simulink model "dronePID"  (R2018b)
settings: Solver=VariableStepAuto  StartTime=0.0  StopTime=10  RelTol=1e-3
libraries: simulink x3
settings Model: Creator=vietdo  LastModifiedBy=Viet Do

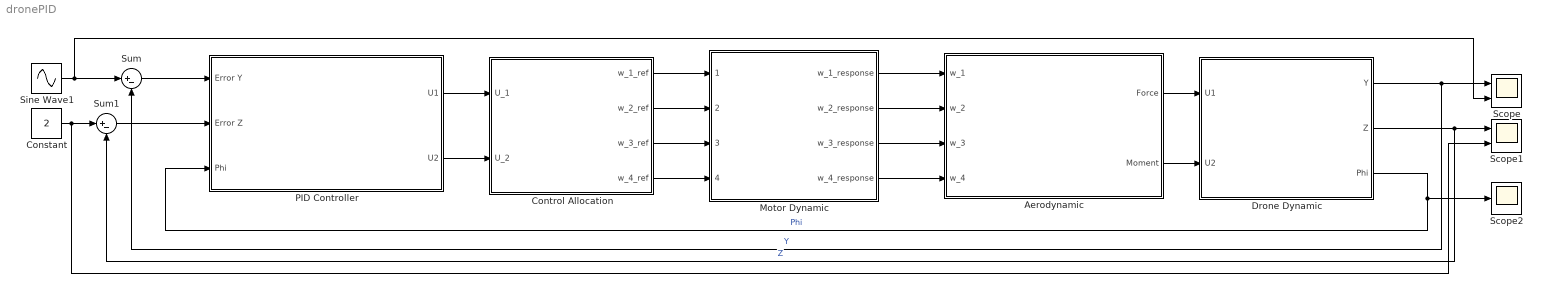
== system dronePID ==
  Aerodynamic : Subsystem  mask{b=2.980e-6, l=0.225}
      mask prompts: b "Lift Constant"; l "Distance between the rotor and the center of mass (m)"
      mask Display: image('blade.png');
  Constant : Constant  Value=2
  Control Allocation : Subsystem  mask{b=2.980e-6, l=0.225}
      mask prompts: b "Lift Constant"; l "Distance between rotor and the center of mass (m)"
      mask Display: image('incsl.png');
  Drone Dynamic : Subsystem  mask{m=0.468, Ixx=4.856e-3, g=9.81}
      mask prompts: m "Mass(kg)"; Ixx "Inertia Moment (kg.m^2)"; g "Gravity(m/s^2)"
      mask Display: image('drone.jpg');
  Motor Dynamic : Subsystem
      mask Display: image('motor.jpg');
  PID Controller : Subsystem
      mask Display: image('PID.png');
  Scope : Scope  NumInputPorts=2
  Scope1 : Scope  NumInputPorts=2
  Scope2 : Scope
  Sine Wave1 : Sin  Frequency=0.2  SampleTime=0
  Sum : Sum  Inputs=|+-
  Sum1 : Sum  Inputs=|+-
  wires:
  Drone Dynamic/1(Y) -> Scope/1, Sum/2  "Y"
  Drone Dynamic/2(Z) -> Scope1/1, Sum1/2  "Z"
  Drone Dynamic/3("Phi ") -> PID Controller/3(Phi), Scope2/1  "Phi"
  Sum/1 -> PID Controller/1(Error Y)
  Sum1/1 -> PID Controller/2(Error Z)
  Sine Wave1/1 -> Scope/2, Sum/1
  Constant/1 -> Scope1/2, Sum1/1
  PID Controller/1(U1) -> Control Allocation/1(U_1)
  PID Controller/2(U2) -> Control Allocation/2(U_2)
  Aerodynamic/1(Force) -> Drone Dynamic/1(U1)
  Aerodynamic/2(Moment) -> Drone Dynamic/2(U2)
  Control Allocation/1(w_1_ref) -> Motor Dynamic/1(1)
  Control Allocation/2(w_2_ref) -> Motor Dynamic/2(2)
  Control Allocation/3(w_3_ref) -> Motor Dynamic/3(3)
  Control Allocation/4(w_4_ref) -> Motor Dynamic/4(4)
  Motor Dynamic/1(w_1_response) -> Aerodynamic/1(w_1)
  Motor Dynamic/2(w_2_response) -> Aerodynamic/2(w_2)
  Motor Dynamic/3(w_3_response) -> Aerodynamic/3(w_3)
  Motor Dynamic/4(w_4_response) -> Aerodynamic/4(w_4)

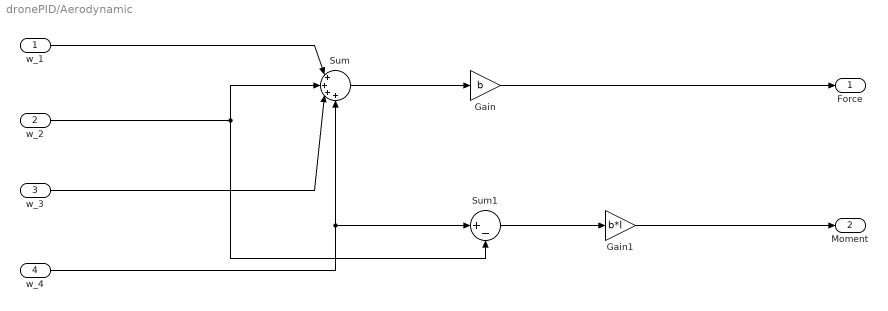
== system dronePID/Aerodynamic ==
  w_1 : Inport
  w_2 : Inport  Port=2
  w_3 : Inport  Port=3
  w_4 : Inport  Port=4
  Gain : Gain  Gain=b
  Gain1 : Gain  Gain=b*l
  Sum : Sum  Inputs=|++++
  Sum1 : Sum  Inputs=|+-
  Force : Outport
  Moment : Outport  Port=2
  wires:
  Sum/1 -> Gain/1
  Gain/1 -> Force/1
  Gain1/1 -> Moment/1
  Sum1/1 -> Gain1/1
  w_1/1 -> Sum/1
  w_2/1 -> Sum1/2, Sum/2
  w_3/1 -> Sum/3
  w_4/1 -> Sum1/1, Sum/4

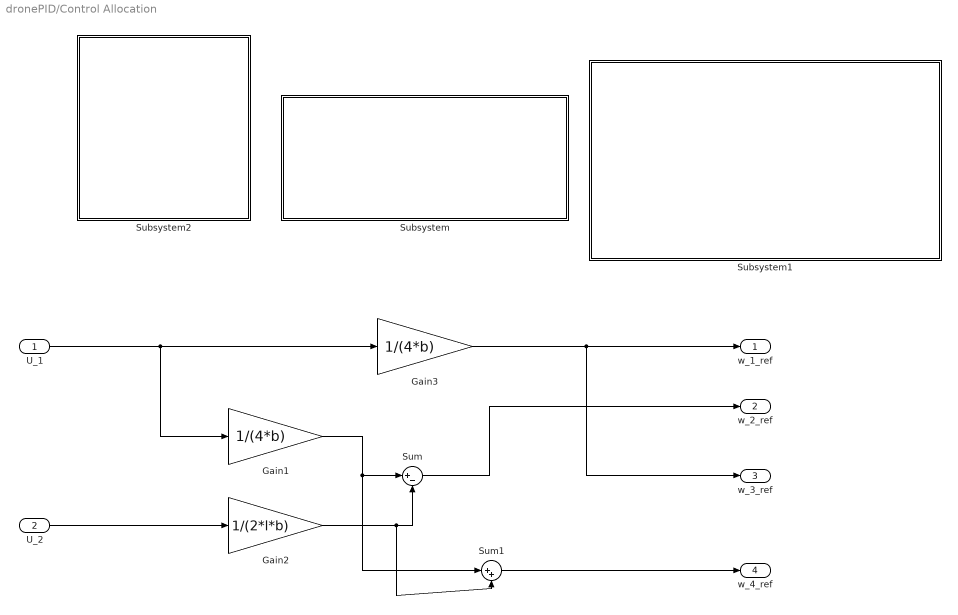
== system dronePID/Control Allocation ==
  U_1 : Inport
  U_2 : Inport  Port=2
  Gain1 : Gain  Gain=1/(4*b)
  Gain2 : Gain  Gain=1/(2*l*b)
  Gain3 : Gain  Gain=1/(4*b)
  Subsystem : Subsystem
      mask Display: image('allocation_1.png');
  Subsystem1 : Subsystem
      mask Display: image('allocation_2.png');
  Subsystem2 : Subsystem
      mask Display: image('allocation_3.png');
  Sum : Sum  Inputs=|+-
  Sum1 : Sum  Inputs=|++
  w_1_ref : Outport
  w_2_ref : Outport  Port=2
  w_3_ref : Outport  Port=3
  w_4_ref : Outport  Port=4
  wires:
  U_1/1 -> Gain3/1, Gain1/1
  Gain1/1 -> Sum1/1, Sum/1
  Gain2/1 -> Sum1/2, Sum/2
  U_2/1 -> Gain2/1
  Gain3/1 -> w_1_ref/1, w_3_ref/1
  Sum/1 -> w_2_ref/1
  Sum1/1 -> w_4_ref/1

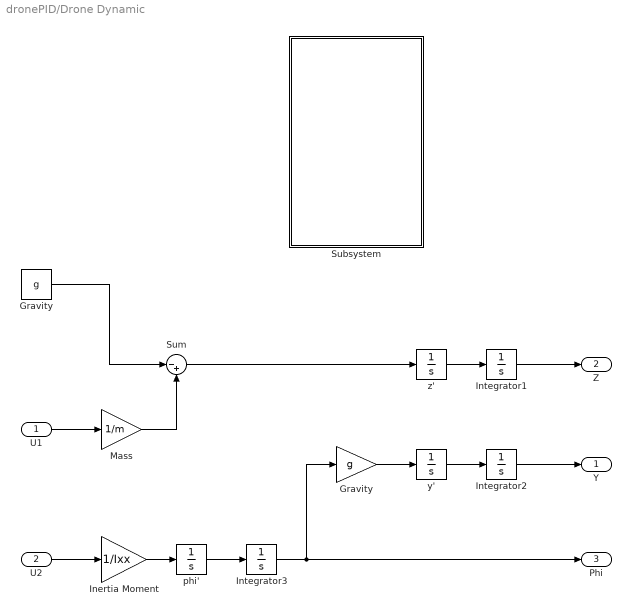
== system dronePID/Drone Dynamic ==
  U1 : Inport
  U2 : Inport  Port=2
  Gravity : Gain  Gain=g
  "Gravity " : Constant  Value=g
  "Inertia Moment " : Gain  Gain=1/Ixx
  Integrator1 : Integrator
  Integrator2 : Integrator
  Integrator3 : Integrator
  "Mass " : Gain  Gain=1/m
  Subsystem : Subsystem
      mask Display: image('dynamic.png');
  Sum : Sum  Inputs=|-+
  phi' : Integrator
  y' : Integrator
  z' : Integrator
  Y : Outport
  Z : Outport  Port=2
  "Phi " : Outport  Port=3
  wires:
  "Gravity "/1 -> Sum/1
  U1/1 -> "Mass "/1
  "Mass "/1 -> Sum/2
  Sum/1 -> z'/1
  z'/1 -> Integrator1/1
  Integrator1/1 -> Z/1
  U2/1 -> "Inertia Moment "/1
  Integrator3/1 -> "Phi "/1, Gravity/1
  "Inertia Moment "/1 -> phi'/1
  phi'/1 -> Integrator3/1
  Integrator2/1 -> Y/1
  Gravity/1 -> y'/1
  y'/1 -> Integrator2/1

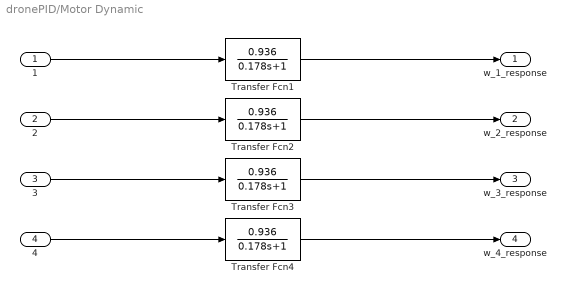
== system dronePID/Motor Dynamic ==
  1 : Inport
  2 : Inport  Port=2
  3 : Inport  Port=3
  4 : Inport  Port=4
  Transfer Fcn{1..4} (4 alike) : TransferFcn  Numerator=[0.936]  Denominator=[0.178 1]
  w_1_response : Outport
  w_2_response : Outport  Port=2
  w_3_response : Outport  Port=3
  w_4_response : Outport  Port=4
  wires:
  Transfer Fcn1/1 -> w_1_response/1
  1/1 -> Transfer Fcn1/1
  4/1 -> Transfer Fcn4/1
  Transfer Fcn4/1 -> w_4_response/1
  Transfer Fcn3/1 -> w_3_response/1
  3/1 -> Transfer Fcn3/1
  Transfer Fcn2/1 -> w_2_response/1
  2/1 -> Transfer Fcn2/1

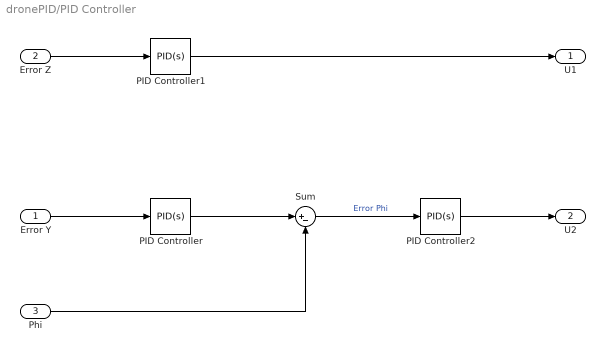
== system dronePID/PID Controller ==
  Error Y : Inport
  Error Z : Inport  Port=2
  Phi : Inport  Port=3
  PID Controller : simulink/Continuous/PID Controller  Controller=PID  Form=Parallel  TimeDomain=Continuous-time  SampleTime=-1  IntegratorMethod=Forward Euler  FilterMethod=Forward Euler  ControllerParametersSource=internal  P=1  I=0  D=0.1  UseFilter=on  N=100  TunerSelectOption=Transfer Function Based (PID Tuner App)  InitialConditionSource=internal  InitialConditionForIntegrator=0  InitialConditionForFilter=0  DifferentiatorICPrevScaledInput=0  ExternalReset=none  TrackingMode=off  Kt=1  LimitOutput=off  UpperSaturationLimit=inf  LowerSaturationLimit=-inf  LinearizeAsGain=on  AntiWindupMode=none  Kb=1  POutMin=[]  POutMax=[]  IOutMin=[]  IOutMax=[]  DOutMin=[]  DOutMax=[]  NOutMin=[]  NOutMax=[]  SumOutMin=[]  SumOutMax=[]  SaturationOutMin=[]  SaturationOutMax=[]  PParamMin=[]  PParamMax=[]  IParamMin=[]  IParamMax=[]  DParamMin=[]  DParamMax=[]  NParamMin=[]  NParamMax=[]  KbParamMin=[]  KbParamMax=[]  KtParamMin=[]  KtParamMax=[]  KbOutMin=[]  KbOutMax=[]  KtOutMin=[]  KtOutMax=[]  IntegratorOutMin=[]  IntegratorOutMax=[]  FilterOutMin=[]  FilterOutMax=[]  SumI1OutMin=[]  SumI1OutMax=[]  SumI2OutMin=[]  SumI2OutMax=[]  SumI3OutMin=[]  SumI3OutMax=[]  SumI4OutMin=[]  SumI4OutMax=[]  SumDOutMin=[]  SumDOutMax=[]  DifferentiatorOutMin=[]  DifferentiatorOutMax=[]  FilterDiffOutCoefMin=[]  FilterDiffOutCoefMax=[]  ReciprocalOutMin=[]  ReciprocalOutMax=[]  SumDenOutMin=[]  SumDenOutMax=[]  SumNumOutMin=[]  SumNumOutMax=[]  DivideOutMin=[]  DivideOutMax=[]  IntegratorContinuousStateAttributes=''  IntegratorStateMustResolveToSignalObject=off  IntegratorRTWStateStorageClass=Auto  FilterContinuousStateAttributes=''  FilterStateMustResolveToSignalObject=off  FilterRTWStateStorageClass=Auto  ParallelPVariant=InternalParameters  IdealPVariant=Disabled  IVariant=InternalParameters  DVariant=InternalParameters  IntegratorVariant=Continuous  SatVariant=Disabled  AWVariant=Passthrough  PCopyVariant=Disabled  TRVariant=Disabled  FdbkBlocksVariant=Forward  IdealPFdbkVariant=Disabled  SatFdbkVariant=Disabled  DerivativeFilterVariant=ContFilter  NVariant=InternalParameters  NCopyVariant=Disabled  FilterICVariant=InternalICsFilter  IntegratorICVariant=InternalICs  ExternalResetVariant=Disabled  TRSumVariant=Passthrough  SumFdbkVariant=Disabled  SumVariant=Sum_PID
  PID Controller1 : simulink/Continuous/PID Controller  Controller=PID  Form=Parallel  TimeDomain=Continuous-time  SampleTime=-1  IntegratorMethod=Forward Euler  FilterMethod=Forward Euler  ControllerParametersSource=internal  P=10  I=2  D=5  UseFilter=on  N=100  TunerSelectOption=Transfer Function Based (PID Tuner App)  InitialConditionSource=internal  InitialConditionForIntegrator=0  InitialConditionForFilter=0  DifferentiatorICPrevScaledInput=0  ExternalReset=none  TrackingMode=off  Kt=1  LimitOutput=off  UpperSaturationLimit=inf  LowerSaturationLimit=-inf  LinearizeAsGain=on  AntiWindupMode=none  Kb=1  POutMin=[]  POutMax=[]  IOutMin=[]  IOutMax=[]  DOutMin=[]  DOutMax=[]  NOutMin=[]  NOutMax=[]  SumOutMin=[]  SumOutMax=[]  SaturationOutMin=[]  SaturationOutMax=[]  PParamMin=[]  PParamMax=[]  IParamMin=[]  IParamMax=[]  DParamMin=[]  DParamMax=[]  NParamMin=[]  NParamMax=[]  KbParamMin=[]  KbParamMax=[]  KtParamMin=[]  KtParamMax=[]  KbOutMin=[]  KbOutMax=[]  KtOutMin=[]  KtOutMax=[]  IntegratorOutMin=[]  IntegratorOutMax=[]  FilterOutMin=[]  FilterOutMax=[]  SumI1OutMin=[]  SumI1OutMax=[]  SumI2OutMin=[]  SumI2OutMax=[]  SumI3OutMin=[]  SumI3OutMax=[]  SumI4OutMin=[]  SumI4OutMax=[]  SumDOutMin=[]  SumDOutMax=[]  DifferentiatorOutMin=[]  DifferentiatorOutMax=[]  FilterDiffOutCoefMin=[]  FilterDiffOutCoefMax=[]  ReciprocalOutMin=[]  ReciprocalOutMax=[]  SumDenOutMin=[]  SumDenOutMax=[]  SumNumOutMin=[]  SumNumOutMax=[]  DivideOutMin=[]  DivideOutMax=[]  IntegratorContinuousStateAttributes=''  IntegratorStateMustResolveToSignalObject=off  IntegratorRTWStateStorageClass=Auto  FilterContinuousStateAttributes=''  FilterStateMustResolveToSignalObject=off  FilterRTWStateStorageClass=Auto  ParallelPVariant=InternalParameters  IdealPVariant=Disabled  IVariant=InternalParameters  DVariant=InternalParameters  IntegratorVariant=Continuous  SatVariant=Disabled  AWVariant=Passthrough  PCopyVariant=Disabled  TRVariant=Disabled  FdbkBlocksVariant=Forward  IdealPFdbkVariant=Disabled  SatFdbkVariant=Disabled  DerivativeFilterVariant=ContFilter  NVariant=InternalParameters  NCopyVariant=Disabled  FilterICVariant=InternalICsFilter  IntegratorICVariant=InternalICs  ExternalResetVariant=Disabled  TRSumVariant=Passthrough  SumFdbkVariant=Disabled  SumVariant=Sum_PID
  PID Controller2 : simulink/Continuous/PID Controller  Controller=PID  Form=Parallel  TimeDomain=Continuous-time  SampleTime=-1  IntegratorMethod=Forward Euler  FilterMethod=Forward Euler  ControllerParametersSource=internal  P=0.1  I=0  D=0.1  UseFilter=on  N=100  TunerSelectOption=Transfer Function Based (PID Tuner App)  InitialConditionSource=internal  InitialConditionForIntegrator=0  InitialConditionForFilter=0  DifferentiatorICPrevScaledInput=0  ExternalReset=none  TrackingMode=off  Kt=1  LimitOutput=off  UpperSaturationLimit=inf  LowerSaturationLimit=-inf  LinearizeAsGain=on  AntiWindupMode=none  Kb=1  POutMin=[]  POutMax=[]  IOutMin=[]  IOutMax=[]  DOutMin=[]  DOutMax=[]  NOutMin=[]  NOutMax=[]  SumOutMin=[]  SumOutMax=[]  SaturationOutMin=[]  SaturationOutMax=[]  PParamMin=[]  PParamMax=[]  IParamMin=[]  IParamMax=[]  DParamMin=[]  DParamMax=[]  NParamMin=[]  NParamMax=[]  KbParamMin=[]  KbParamMax=[]  KtParamMin=[]  KtParamMax=[]  KbOutMin=[]  KbOutMax=[]  KtOutMin=[]  KtOutMax=[]  IntegratorOutMin=[]  IntegratorOutMax=[]  FilterOutMin=[]  FilterOutMax=[]  SumI1OutMin=[]  SumI1OutMax=[]  SumI2OutMin=[]  SumI2OutMax=[]  SumI3OutMin=[]  SumI3OutMax=[]  SumI4OutMin=[]  SumI4OutMax=[]  SumDOutMin=[]  SumDOutMax=[]  DifferentiatorOutMin=[]  DifferentiatorOutMax=[]  FilterDiffOutCoefMin=[]  FilterDiffOutCoefMax=[]  ReciprocalOutMin=[]  ReciprocalOutMax=[]  SumDenOutMin=[]  SumDenOutMax=[]  SumNumOutMin=[]  SumNumOutMax=[]  DivideOutMin=[]  DivideOutMax=[]  IntegratorContinuousStateAttributes=''  IntegratorStateMustResolveToSignalObject=off  IntegratorRTWStateStorageClass=Auto  FilterContinuousStateAttributes=''  FilterStateMustResolveToSignalObject=off  FilterRTWStateStorageClass=Auto  ParallelPVariant=InternalParameters  IdealPVariant=Disabled  IVariant=InternalParameters  DVariant=InternalParameters  IntegratorVariant=Continuous  SatVariant=Disabled  AWVariant=Passthrough  PCopyVariant=Disabled  TRVariant=Disabled  FdbkBlocksVariant=Forward  IdealPFdbkVariant=Disabled  SatFdbkVariant=Disabled  DerivativeFilterVariant=ContFilter  NVariant=InternalParameters  NCopyVariant=Disabled  FilterICVariant=InternalICsFilter  IntegratorICVariant=InternalICs  ExternalResetVariant=Disabled  TRSumVariant=Passthrough  SumFdbkVariant=Disabled  SumVariant=Sum_PID
  Sum : Sum  Inputs=|+-
  U1 : Outport
  U2 : Outport  Port=2
  wires:
  Error Y/1 -> PID Controller/1
  Error Z/1 -> PID Controller1/1
  Phi/1 -> Sum/2
  PID Controller/1 -> Sum/1
  Sum/1 -> PID Controller2/1  "Error Phi"
  PID Controller2/1 -> U2/1
  PID Controller1/1 -> U1/1

== system dronePID/Control Allocation/Subsystem ==

== system dronePID/Control Allocation/Subsystem1 ==

== system dronePID/Control Allocation/Subsystem2 ==

== system dronePID/Drone Dynamic/Subsystem ==
